simulink library "multiSpoolingController_ul"  (R2018b)
settings: Solver=VariableStepAuto  StartTime=0.0  StopTime=10.0  RelTol=1e-3
undefined symbols (not defined in the file or in its folder): pathCtrl
libraries: firstOrderFilter_ul x1
settings Model: Creator=James Reed  LastModifiedBy=mcobb

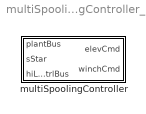
== system multiSpoolingController_ul ==
  multiSpoolingController : Subsystem

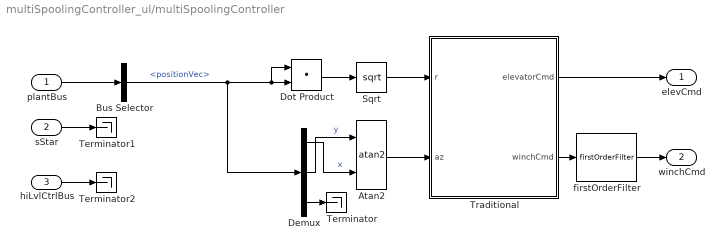
== system multiSpoolingController_ul/multiSpoolingController ==
  "plantBus " : Inport  OutDataTypeStr=Bus: plantBus
  "sStar " : Inport  Port=2
  hiLvlCtrlBus : Inport  Port=3  OutDataTypeStr=Bus: hiLvlCtrlBus
  Atan2 : Trigonometry  Operator=atan2
  Bus Selector : BusSelector  OutputSignals=positionVec
  Demux : Demux  Outputs=3
  Dot Product : DotProduct  InputSameDT=on  OutDataTypeStr=Inherit: Inherit via internal rule
  Sqrt : Sqrt  SaturateOnIntegerOverflow=on
  Terminator : Terminator
  Terminator1 : Terminator
  Terminator2 : Terminator
  Traditional : Stateflow chart  TreatAsAtomicUnit=on  mask{maxR=pathCtrl.maxR.Value, minR=pathCtrl.minR.Value, winchSpeedIn=pathCtrl.winchSpeedIn.Value, winchSpeedOut=pathCtrl.winchSpeedOut.Value, elevatorReelInDef=pathCtrl.elevatorReelInDef.Value}
      mask prompts: maxR "Min tether length"; minR "Max tether length"; winchSpeedIn "Spool in speed"; winchSpeedOut "Spool out speed"; elevatorReelInDef "Elevator deflection during spool in"
  firstOrderFilter : firstOrderFilter_ul/firstOrderFilter  tau=1  ic=0
  elevCmd : Outport
  "winchCmd " : Outport  Port=2
  wires:
  Traditional/1(elevatorCmd) -> elevCmd/1
  Traditional/2(winchCmd) -> firstOrderFilter/1
  firstOrderFilter/1 -> "winchCmd "/1
  Bus Selector/1 -> Dot Product/2, Dot Product/1, Demux/1  "<positionVec>"
  "sStar "/1 -> Terminator1/1
  Demux/3 -> Terminator/1
  Sqrt/1 -> Traditional/1(r)
  Atan2/1 -> Traditional/2(az)
  Demux/1 -> Atan2/2  "x"
  Demux/2 -> Atan2/1  "y"
  Dot Product/1 -> Sqrt/1
  "plantBus "/1 -> Bus Selector/1
  hiLvlCtrlBus/1 -> Terminator2/1

== stateflow chart multiSpoolingController_ul/multiSpoolingController/Traditional ==
  state SpoolOut
    entry:
    winchCmd = winchSpeedOut;
    elevatorCmd = 0;
  state SpoolIn
    winchCmd = winchSpeedIn;
    elevatorCmd = elevatorReelInDef;
  (default) -> SpoolIn
  SpoolOut -> SpoolIn : [r > maxR ]
  SpoolIn -> SpoolOut : [r < minR]
  data: elevatorCmd output; r input; az input; winchCmd output; elevatorReelInDef parameter; winchSpeedOut parameter; winchSpeedIn parameter; minR parameter; maxR parameter
